simulink model "kinect1_code"  (R2015a)
settings: Solver=ode45  StartTime=0.0  StopTime=10.0  RelTol=1e-3
libraries: robotlib x4
settings Model: Creator=trandh  LastModifiedBy=trandh

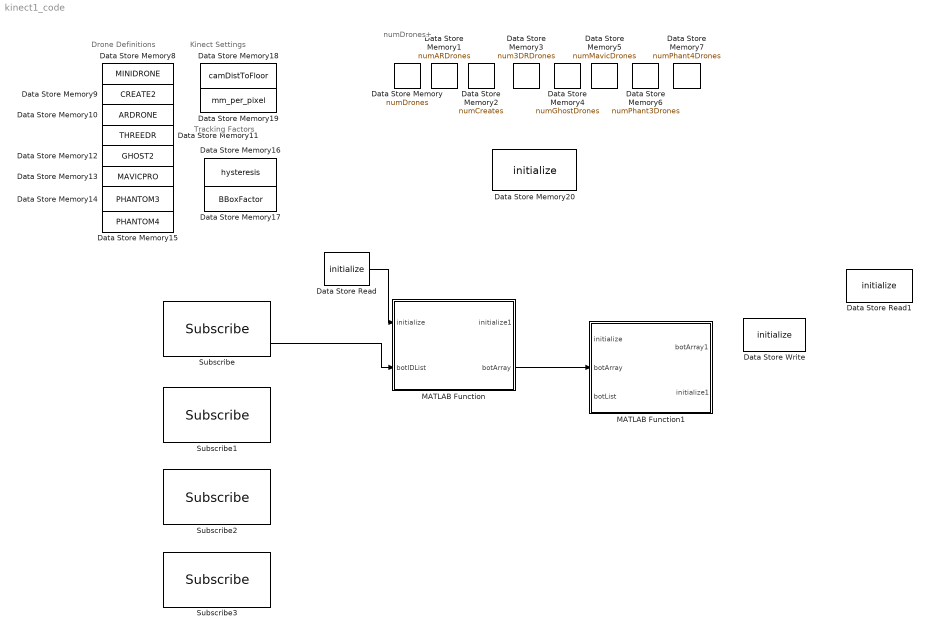
== system kinect1_code ==
  note: numDrones+
  note: Tracking Factors
  note: Kinect Settings
  note: Drone Definitions
  Data Store Memory : DataStoreMemory  DataStoreName=numDrones  ReadBeforeWriteMsg=warning  WriteAfterWriteMsg=warning  WriteAfterReadMsg=warning
  Data Store Memory1 : DataStoreMemory  DataStoreName=numARDrones  ReadBeforeWriteMsg=warning  WriteAfterWriteMsg=warning  WriteAfterReadMsg=warning
  Data Store Memory10 : DataStoreMemory  DataStoreName=ARDRONE  ReadBeforeWriteMsg=warning  WriteAfterWriteMsg=warning  WriteAfterReadMsg=warning  InitialValue=102
  Data Store Memory11 : DataStoreMemory  DataStoreName=THREEDR  ReadBeforeWriteMsg=warning  WriteAfterWriteMsg=warning  WriteAfterReadMsg=warning  InitialValue=103
  Data Store Memory12 : DataStoreMemory  DataStoreName=GHOST2  ReadBeforeWriteMsg=warning  WriteAfterWriteMsg=warning  WriteAfterReadMsg=warning  InitialValue=104
  Data Store Memory13 : DataStoreMemory  DataStoreName=MAVICPRO  ReadBeforeWriteMsg=warning  WriteAfterWriteMsg=warning  WriteAfterReadMsg=warning  InitialValue=105
  Data Store Memory14 : DataStoreMemory  DataStoreName=PHANTOM3  ReadBeforeWriteMsg=warning  WriteAfterWriteMsg=warning  WriteAfterReadMsg=warning  InitialValue=106
  Data Store Memory15 : DataStoreMemory  DataStoreName=PHANTOM4  ReadBeforeWriteMsg=warning  WriteAfterWriteMsg=warning  WriteAfterReadMsg=warning  InitialValue=107
  Data Store Memory16 : DataStoreMemory  DataStoreName=hysteresis  ReadBeforeWriteMsg=warning  WriteAfterWriteMsg=warning  WriteAfterReadMsg=warning  InitialValue=1000
  Data Store Memory17 : DataStoreMemory  DataStoreName=BBoxFactor  ReadBeforeWriteMsg=warning  WriteAfterWriteMsg=warning  WriteAfterReadMsg=warning  InitialValue=1.5
  Data Store Memory18 : DataStoreMemory  DataStoreName=camDistToFloor  ReadBeforeWriteMsg=warning  WriteAfterWriteMsg=warning  WriteAfterReadMsg=warning  InitialValue=3058
  Data Store Memory19 : DataStoreMemory  DataStoreName=mm_per_pixel  ReadBeforeWriteMsg=warning  WriteAfterWriteMsg=warning  WriteAfterReadMsg=warning  InitialValue=5.663295322
  Data Store Memory2 : DataStoreMemory  DataStoreName=numCreates  ReadBeforeWriteMsg=warning  WriteAfterWriteMsg=warning  WriteAfterReadMsg=warning
  Data Store Memory20 : DataStoreMemory  DataStoreName=initialize  ReadBeforeWriteMsg=warning  WriteAfterWriteMsg=warning  WriteAfterReadMsg=warning  InitialValue=1
  Data Store Memory3 : DataStoreMemory  DataStoreName=num3DRDrones  ReadBeforeWriteMsg=warning  WriteAfterWriteMsg=warning  WriteAfterReadMsg=warning
  Data Store Memory4 : DataStoreMemory  DataStoreName=numGhostDrones  ReadBeforeWriteMsg=warning  WriteAfterWriteMsg=warning  WriteAfterReadMsg=warning
  Data Store Memory5 : DataStoreMemory  DataStoreName=numMavicDrones  ReadBeforeWriteMsg=warning  WriteAfterWriteMsg=warning  WriteAfterReadMsg=warning
  Data Store Memory6 : DataStoreMemory  DataStoreName=numPhant3Drones  ReadBeforeWriteMsg=warning  WriteAfterWriteMsg=warning  WriteAfterReadMsg=warning
  Data Store Memory7 : DataStoreMemory  DataStoreName=numPhant4Drones  ReadBeforeWriteMsg=warning  WriteAfterWriteMsg=warning  WriteAfterReadMsg=warning
  Data Store Memory8 : DataStoreMemory  DataStoreName=MINIDRONE  ReadBeforeWriteMsg=warning  WriteAfterWriteMsg=warning  WriteAfterReadMsg=warning  InitialValue=100
  Data Store Memory9 : DataStoreMemory  DataStoreName=CREATE2  ReadBeforeWriteMsg=warning  WriteAfterWriteMsg=warning  WriteAfterReadMsg=warning  InitialValue=101
  Data Store Read : DataStoreRead  DataStoreName=initialize
  Data Store Read1 : DataStoreRead  DataStoreName=initialize
  Data Store Write : DataStoreWrite  DataStoreName=initialize
  MATLAB Function : MATLAB Function  TreatAsAtomicUnit=on
  MATLAB Function1 : MATLAB Function  TreatAsAtomicUnit=on
  Subscribe : robotlib/Subscribe  SourceLibraryInfo=This block requires Robotics System Toolbox  topicSource=Specify your own  topic=/botID_list  messageType=std_msgs/String  sampleTime=-1  messageQueueLength=1
  Subscribe1 : robotlib/Subscribe  SourceLibraryInfo=This block requires Robotics System Toolbox  topicSource=Specify your own  topic=/kinect1/bot_list  messageType=std_msgs/String  sampleTime=-1  messageQueueLength=1
  Subscribe2 : robotlib/Subscribe  SourceLibraryInfo=This block requires Robotics System Toolbox  topicSource=Specify your own  topic=/kinect1/incomming  messageType=geometry_msgs/Point  sampleTime=-1  messageQueueLength=1
  Subscribe3 : robotlib/Subscribe  SourceLibraryInfo=This block requires Robotics System Toolbox  topicSource=Specify your own  topic=/window_command  messageType=std_msgs/String  sampleTime=-1  messageQueueLength=1
  wires:
  Subscribe/2 -> MATLAB Function/2(botIDList)
  MATLAB Function/2(botArray) -> MATLAB Function1/2(botArray)
  Data Store Read/1 -> MATLAB Function/1(initialize)

== matlab function kinect1_code/MATLAB Function1 ==
  data: initialize input; botArray input; botList input; mm_per_pixel data_store_memory; camDistToFloor data_store_memory; BBoxFactor data_store_memory; hysteresis data_store_memory; MINIDRONE data_store_memory; CREATE2 data_store_memory; ARDRONE data_store_memory; THREEDR data_store_memory; GHOST2 data_store_memory; MAVICPRO data_store_memory; PHANTOM3 data_store_memory; PHANTOM4 data_store_memory; botArray1 output; initialize1 output
function [botArray1, initialize1] = find_bots(initialize, botArray, botList) 
%#codegen
% Author: Nathaniel Hamilton
%  Email: nathaniel.p.hamilton@vanderbilt.edu
%
% Purpose: Find all the bots in their initial position and identify them

% Declare global variables that will be used or defined
global mm_per_pixel
global camDistToFloor
global BBoxFactor
global hysteresis
global MINIDRONE
global CREATE2
global ARDRONE
global THREEDR
global GHOST2
global MAVICPRO
global PHANTOM3
global PHANTOM4

% If this isn't the first call, don't do anything
if initialize == 0
    return;
end

% turn the botList from a string to a listof integers
specificList = str2num(botList);
robot_count = length(specificList);

% Determine the number of each type of robot present
numDrones = 0;
numCreates = 0;
numARDrones = 0;
num3DRDrones = 0;
numGhostDrones = 0;
numMavicDrones = 0;
numPhant3Drones = 0;
numPhant4Drones = 0;
for i = specificList
    currentType = botArray(i).type;
    if currentType == MINIDRONE
        numDrones = numDrones + 1;
    elseif currentType == CREATE2
        numCreates = numCreates + 1;
    elseif currentType == ARDRONE
        numARDrones = numARDrones + 1;
    elseif currentType == THREEDR
        num3DRDrones = num3DRDrones + 1;
    elseif currentType == GHOST2
        numGhostDrones = numGhostDrones + 1;
    elseif currentType == MAVICPRO
        numMavicDrones = numMavicDrones + 1;
    elseif currentType == PHANTOM3
        numPhant3Drones = numPhant3Drones + 1;
    elseif currentType == PHANTOM4
        numPhant4Drones = numPhant4Drones + 1;
    end
end

% Run findBots to find all the bots and then assign their names
found = false;
while ~found
    trigger([vid vid2])
    % Get the acquired frames and metadata.
    [imgColor, ts_color, metaData_Color] = getdata(vid);
    [imgDepth, ts_depth, metaData_Depth] = getdata(vid2);
    % make this function modify botArray, instead of return so many things
    [found, bots] = findBots(imgColor, imgDepth, numDrones, numCreates, ...
        numARDrones, num3DRDrones, numGhostDrones, numMavicDrones, ...
        numPhant3Drones, numPhant4Drones); %HEY THIS NEEDS TO BE MADE
end

% Match each robot found to it's designated name
for i = specificList
    k = 1;
    while k < robot_count
        if botArray(i).type == bots(k).type
            if botArray(i).color == bots(k).color
                % If the type and color match, then the robot name
                % is given to that robot
                botArray(i) = bots(k);
                break;
            else
                k = k + 1;
            end
        else
            k = k + 1;
        end
    end
end

return;

== matlab function kinect1_code/MATLAB Function ==
  data: initialize1 output; initialize input; botIDList input; botArray output; mm_per_pixel data_store_memory; camDistToFloor data_store_memory; BBoxFactor data_store_memory; hysteresis data_store_memory; MINIDRONE data_store_memory; CREATE2 data_store_memory; ARDRONE data_store_memory; THREEDR data_store_memory; GHOST2 data_store_memory; MAVICPRO data_store_memory; PHANTOM3 data_store_memory; PHANTOM4 data_store_memory
function [initialize1, botArray] = initialize_system(initialize, botIDList)
%#codegen
% Author: Nathaniel Hamilton
%  Email: nathaniel.p.hamilton@vanderbilt.edu
%
% Purpose: The purpose of this function is to gether information from the
% master about how many bots there are in the system and, more
% specifically, which ones need to be found at this node. Additionally, the
% Kinect is initialized in this function.

% Declare global variables that will be used or defined
global mm_per_pixel
global camDistToFloor
global BBoxFactor
global hysteresis
global MINIDRONE
global CREATE2
global ARDRONE
global THREEDR
global GHOST2
global MAVICPRO
global PHANTOM3
global PHANTOM4

% Drone definitions
MINIDRONE = 100;
CREATE2 = 101;
ARDRONE = 102;
THREEDR = 103;
GHOST2 = 104;
MAVICPRO = 105;
PHANTOM3 = 106;
PHANTOM4 = 107;

% Kinect Settings
camDistToFloor = 3058; % in mm, as measured with Kinect
mm_per_pixel = 5.663295322; % mm in one pixel at ground level
warning('off','images:imfindcircles:warnForSmallRadius')

% Tracking Factors
hysteresis = 100;
BBoxFactor = 1.7;

% Initialize botArray and assign all bots to their location
splitBotList = strsplit(botIDList, ','); %HEY NATE THIS THING MIGHT BE DIFFERENT!!!
robot_count = length(splitBotList);
robNames = cell(1,robot_count);
robTypes = cell(1,robot_count);
robColors = cell(1,robot_count);

for i = 1:robot_count
    currentRobInfo = strsplit(splitBotList(i));
    robNames(i) = currentRobInfo(1);
    robTypes(i) = currentRobInfo(2);
    robColors(i) = currentRobInfo(3);
end

botArray = Robot.empty(robot_count,0);
for i = 1:robot_count
    botArray(i) = Robot;
    botArray(i).name = robNames(i);
    botArray(i).type = robTypes(i);
    botArray(i).color = robColors(i);
end


% Initialize the Kinect by capturing a few frames
if exist('vid', 'var') && exist('vid2', 'var')
    stop([vid vid2]);
    clear vid vid2;
elseif exist('vid1', 'var') && exist('vid2', 'var')
    stop([vid1 vid2]);
    clear vid1 vid2;
end

vid1 = videoinput('kinect',1); %color 
vid2 = videoinput('kinect',2); %depth

vid1.FramesPerTrigger = 1;
vid2.FramesPerTrigger = 1;

vid1.TriggerRepeat = num_frames;
vid2.TriggerRepeat = num_frames;

triggerconfig([vid1 vid2],'manual');
start([vid1 vid2]);
% trigger a couple times in case first frames are bad
trigger([vid1 vid2])
trigger([vid1 vid2]) 


return;
